simulink model "rluav"  (R2022b)
settings: Solver=ode45  StartTime=0.0  StopTime=200.0  FixedStep=Ts  RelTol=1e-3  EnableMultiTasking=on
values from neighbouring files (symbols this model uses):
  Ts = 1/50.0    (= 0.02)    [rluav_init.m]
undefined symbols (not defined in the file or in its folder): DiscIntNeverNeededParam
libraries: simulink x5, rllib x1
settings Model: Creator=The MathWorks, Inc.  LastModifiedBy=csu405
settings SolverCC: AlgebraicLoopSolver=TrustRegion
settings DataIOCC: LimitDataPoints=on  SaveFormat=Array  ReturnWorkspaceOutputs=off  SignalLoggingName=logsOut
settings OptimizationCC: ExpressionDepthLimit=2147483647  InitFltsAndDblsToZero=on  LifeSpan=inf
settings DebuggingCC: SaveWithParameterizedLinksMsg=none  UnderspecifiedInitializationDetection=Classic  MergeDetectMultiDrivingBlocksExec=none  SignalResolutionControl=TryResolveAllWithWarning  MultiTaskDSMMsg=warning  FcnCallInpInsideContextMsg=warning  UnconnectedInputMsg=warning  UnconnectedOutputMsg=warning  UnconnectedLineMsg=warning  AllowSymbolicDim=off  StateNameClashWarn=warning  SFUnexpectedBacktrackingDiag=warning  SFNoUnconditionalDefaultTransitionDiag=warning  SFExecutionAtInitializationDiag=none  SFMachineParentedDataDiag=warning  ArithmeticOperatorsInVariantConditions=warning
settings HardwareCC: ProdBitPerPointer=32  ProdBitPerSizeT=32  ProdBitPerPtrDiffT=32  ProdLargestAtomicFloat=None  ProdIntDivRoundTo=Undefined  ProdEndianess=Unspecified  ProdWordSize=32  ProdHWDeviceType=Specified
settings ModelReferenceCC: EnableRefExpFcnMdlSchedulingChecks=on  PropagateSignalLabelsOutOfModel=off
settings SFSimCC: SimUseLocalCustomCode=off
settings RTWCC: RTWUseLocalCustomCode=off
settings CodeAppCC: StateflowObjectComments=on
settings GRTTargetCC: TargetFcnLib=ansi_tfl_tmw.mat  TargetLangStandard=C89/C90 (ANSI)  CombineOutputUpdateFcns=off  GRTInterface=on
settings ConfigComp: CovMetricSettings=dw  CovSaveCumulativeToWorkspaceVar=on  CovSaveSingleToWorkspaceVar=on  CovExternalEMLEnable=off

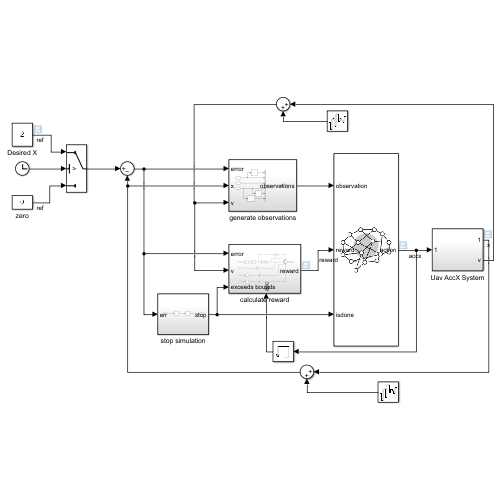
[thumbnail: Simulink's stored preview of the top-level diagram]
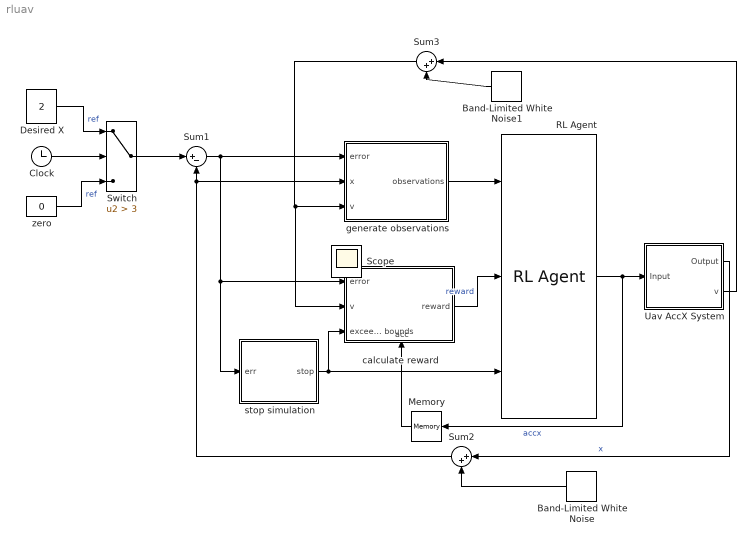
== system rluav ==
  Band-Limited White Noise : simulink/Sources/Band-Limited White Noise  Cov=[0.002]  Ts=Ts  seed=[23341]
  Band-Limited White Noise1 : simulink/Sources/Band-Limited White Noise  Cov=[0.002]  Ts=Ts  seed=[23341]
  Clock : Clock
  Desired X : Constant  Value=2
  Memory : Memory
  RL Agent : rllib/RL Agent  Agent=agent  ExternalActionAsInput=off  ProvideLastAction=off  ProvideCumRwd=off  TreatAsDirectFeedthrough=on  UseStrictObservationDataTypes=off
  Sum1 : Sum  Inputs=|+-  SaturateOnIntegerOverflow=on
  Sum2 : Sum  Inputs=|++  SaturateOnIntegerOverflow=on
  Sum3 : Sum  Inputs=|++  SaturateOnIntegerOverflow=on
  Switch : Switch  Criteria=u2 > Threshold  Threshold=3  SaturateOnIntegerOverflow=off  InputSameDT=off
  Uav AccX System : Subsystem
  calculate reward : Subsystem
      settings: PortSchema="{\"entries\":[{\"content\":{\"sides\":[{\"content\":{\"connectorIds\":[\"In1\",\"In2\",\"In3\"]},\"type\":\"ConnectorPlacement.EquallySpacedRectSide\",\"uuid\":\"a6831b4c-c5e4-4b81-8e40-7fc4b7dad633\"},{\"content\":{\"connectorIds\":[\"Out1\"],\"side\":\"RIGHT\"},\"type\":\"ConnectorPlacement.EquallySpacedRectSide\",\"uuid\":\"8e922aec-ef45-4070-9445-bf1f36bf8a17\"},{\"content\":{\"connectorIds\":[],\"side\":\"TOP\"},\"type\":\"ConnectorPlacement.EquallySpacedRectSide\",\"uuid\":\"70fa4f95-2353-478a-a00d-3d58ec9167ce\"},{\"content\":{\"connectorIds\":[\"In4\"],\"side\":\"BOTTOM\"},\"type\":\"ConnectorPlacement.EquallySpacedRectSide\",\"uuid\":\"92073c7e-e113-4538-8fec-17539d6aadbe\"}]},\"type\":\"ConnectorPlacement.EquallySpacedConnector\",\"uuid\":\"a5a5b4e0-4f16-4179-a493-15187e3b2ccc\"}],\"packageUris\":[\"http://schema.mathworks.com/mf0/Connector/R2020b\"],\"version\":\"1.0\"}"
  generate observations : Subsystem
  stop simulation : Subsystem
  zero : Constant  Value=0
  Scope : Scope
  wires:
  Sum1/1 -> generate observations/1(error), stop simulation/1(err), calculate reward/1(error)
  RL Agent/1 -> Memory/1, Uav AccX System/1(Input)  "accx"
  stop simulation/1(stop) -> calculate reward/3(exceeds bounds), RL Agent/3
  calculate reward/1(reward) -> RL Agent/2  "reward"
  generate observations/1(observations) -> RL Agent/1
  Band-Limited White Noise/1 -> Sum2/2
  Uav AccX System/1(Output) -> Sum2/1  "x"
  Sum2/1 -> generate observations/2(x), Sum1/2
  Uav AccX System/2(v) -> Sum3/1
  Band-Limited White Noise1/1 -> Sum3/2
  Sum3/1 -> calculate reward/2(v), generate observations/3(v)
  Memory/1 -> calculate reward/4(acc)
  Desired X/1 -> Switch/1  "ref"
  Switch/1 -> Sum1/1
  Clock/1 -> Switch/2
  zero/1 -> Switch/3  "ref"

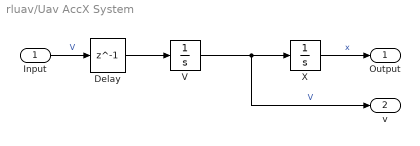
== system rluav/Uav AccX System ==
  Input : Inport
  Delay : Delay  DelayLength=1  InitialCondition=0
  V : Integrator  LimitOutput=on  UpperSaturationLimit=100  LowerSaturationLimit=-100
  X : Integrator  LimitOutput=on  UpperSaturationLimit=100  LowerSaturationLimit=-100
  Output : Outport  VectorParamsAs1DForOutWhenUnconnected=off
  v : Outport  Port=2  VectorParamsAs1DForOutWhenUnconnected=off
  wires:
  Input/1 -> Delay/1  "V"
  X/1 -> Output/1  "x"
  V/1 -> X/1, v/1  "V"
  Delay/1 -> V/1

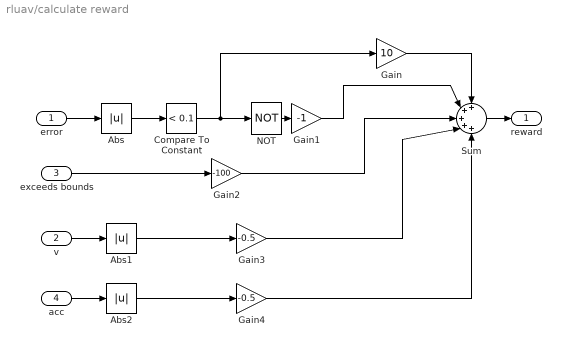
== system rluav/calculate reward ==
  error : Inport
  v : Inport  Port=2
  exceeds bounds : Inport  Port=3
  acc : Inport  Port=4
  Abs : Abs  SaturateOnIntegerOverflow=off
  Abs1 : Abs  ZeroCross=off  SaturateOnIntegerOverflow=off
  Abs2 : Abs  ZeroCross=off  SaturateOnIntegerOverflow=off
  Compare To Constant : simulink/Logic and Bit Operations/Compare To Constant  relop=<  const=0.1  OutDataTypeStr=boolean
  Gain : Gain  Gain=10
  Gain1 : Gain  Gain=-1
  Gain2 : Gain  Gain=-100
  Gain3 : Gain  Gain=-0.5
  Gain4 : Gain  Gain=-0.5
  NOT : Logic  Operator=NOT  IconShape=distinctive  AllPortsSameDT=off  OutDataTypeStr=boolean
  Sum : Sum  Inputs=+++++  OutDataTypeStr=double
  reward : Outport  VectorParamsAs1DForOutWhenUnconnected=off
  wires:
  Abs/1 -> Compare To Constant/1
  Gain2/1 -> Sum/3
  Gain/1 -> Sum/1
  Compare To Constant/1 -> NOT/1, Gain/1
  Gain1/1 -> Sum/2
  Sum/1 -> reward/1
  NOT/1 -> Gain1/1
  exceeds bounds/1 -> Gain2/1
  error/1 -> Abs/1
  v/1 -> Abs1/1
  Gain3/1 -> Sum/4
  Abs1/1 -> Gain3/1
  Abs2/1 -> Gain4/1
  acc/1 -> Abs2/1
  Gain4/1 -> Sum/5

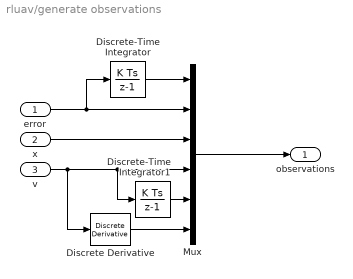
== system rluav/generate observations ==
  error : Inport
  x : Inport  Port=2
  v : Inport  Port=3
  Discrete Derivative : simulink/Discrete/Discrete Derivative  gainval=0.01  ICPrevScaledInput=0.0  OutMin=[]  OutMax=[]  OutDataType=fixdt(1, 16)  OutScaling=2^-10  DoSatur=off
  Discrete-Time Integrator : DiscreteIntegrator  SampleTime=Ts  ICPrevOutput=DiscIntNeverNeededParam  ICPrevScaledInput=DiscIntNeverNeededParam
  Discrete-Time Integrator1 : DiscreteIntegrator  gainval=0.1  SampleTime=Ts  ICPrevOutput=DiscIntNeverNeededParam  ICPrevScaledInput=DiscIntNeverNeededParam
  Mux : Mux  Inputs=6
  observations : Outport  VectorParamsAs1DForOutWhenUnconnected=off
  wires:
  x/1 -> Mux/3
  Discrete-Time Integrator/1 -> Mux/1
  error/1 -> Discrete-Time Integrator/1, Mux/2
  Mux/1 -> observations/1
  v/1 -> Discrete Derivative/1, Discrete-Time Integrator1/1, Mux/4
  Discrete-Time Integrator1/1 -> Mux/5
  Discrete Derivative/1 -> Mux/6

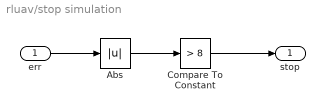
== system rluav/stop simulation ==
  err : Inport
  Abs : Abs  SaturateOnIntegerOverflow=off
  Compare To Constant : simulink/Logic and Bit Operations/Compare To Constant  relop=>  const=8  OutDataTypeStr=boolean
  stop : Outport  VectorParamsAs1DForOutWhenUnconnected=off
  wires:
  err/1 -> Abs/1
  Abs/1 -> Compare To Constant/1
  Compare To Constant/1 -> stop/1
